simulink model "alloc_couple"  (R2024b)
settings: Solver=FixedStepAuto  StartTime=0.0  StopTime=5  RelTol=1e-3
values from neighbouring files (symbols this model uses):
  r_wheels = 0.470/2    (= 0.235)    [main_phi.m]
  tr = 1.2    [main_phi.m]
settings Model: Creator=marti  LastModifiedBy=marti

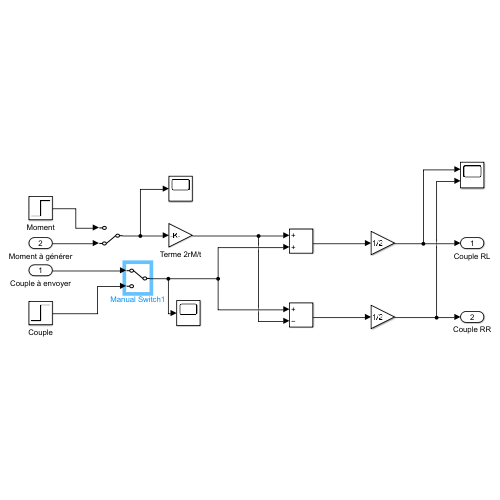
[thumbnail: Simulink's stored preview of the top-level diagram]
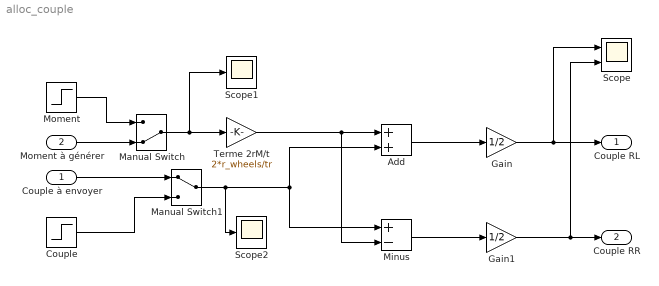
== system alloc_couple ==
  Couple à envoyer : Inport
  Moment à générer : Inport  Port=2
  Add : Sum
  Couple : Step  Time=0  After=300  SampleTime=0
  Gain : Gain  Gain=1/2
  Gain1 : Gain  Gain=1/2
  Manual Switch : ManualSwitch  CurrentSetting=0
  Manual Switch1 : ManualSwitch
  Minus : Sum  Inputs=+-
  Moment : Step  After=50  SampleTime=0
  Scope : Scope  NumInputPorts=2
  Scope1 : Scope
  Scope2 : Scope
  Terme 2rM/t : Gain  Gain=2*r_wheels/tr
  Couple RL : Outport
  Couple RR : Outport  Port=2
  wires:
  Terme 2rM/t/1 -> Minus/2, Add/1
  Add/1 -> Gain/1
  Minus/1 -> Gain1/1
  Gain1/1 -> Scope/2, Couple RR/1
  Gain/1 -> Scope/1, Couple RL/1
  Manual Switch/1 -> Scope1/1, Terme 2rM/t/1
  Moment à générer/1 -> Manual Switch/2
  Moment/1 -> Manual Switch/1
  Manual Switch1/1 -> Scope2/1, Minus/1, Add/2
  Couple à envoyer/1 -> Manual Switch1/1
  Couple/1 -> Manual Switch1/2
